simulink model "cntrl2"  (R2013a)
settings: Solver=ode45  StartTime=0.0  StopTime=20  RelTol=1e-3
undefined symbols (not defined in the file): C, G, H, K, L1
settings Model: Creator=Daniel  LastModifiedBy=Daniel

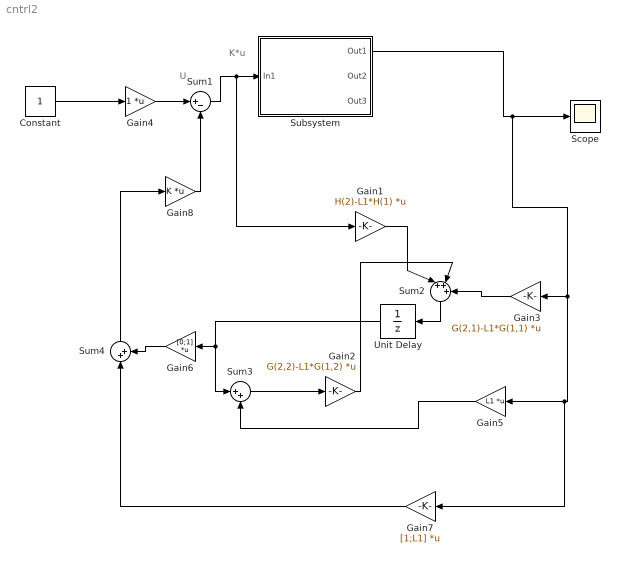
== system cntrl2 ==
  note: U
  note: K*u
  Constant : Constant
  Gain1 : Gain  Gain=H(2)-L1*H(1)  Multiplication=Matrix(K*u) (u vector)
  Gain2 : Gain  Gain=G(2,2)-L1*G(1,2)  Multiplication=Matrix(K*u) (u vector)
  Gain3 : Gain  Gain=G(2,1)-L1*G(1,1)  Multiplication=Matrix(K*u) (u vector)
  Gain4 : Gain  Multiplication=Matrix(K*u) (u vector)
  Gain5 : Gain  Gain=L1  Multiplication=Matrix(K*u) (u vector)
  Gain6 : Gain  Gain=[0;1]  Multiplication=Matrix(K*u) (u vector)
  Gain7 : Gain  Gain=[1;L1]  Multiplication=Matrix(K*u) (u vector)
  Gain8 : Gain  Gain=K  Multiplication=Matrix(K*u) (u vector)
  Scope : Scope
  Subsystem : Subsystem
      mask Display: image('b747.jpg')
  Sum1 : Sum  Inputs=|+-
  Sum2 : Sum  Inputs=|+++
  Sum3 : Sum  Inputs=|++
  Sum4 : Sum  Inputs=|++
  Unit Delay : UnitDelay  InitialCondition=4
  wires:
  Sum1/1 -> Gain1/1, Subsystem/1(In1)
  Gain4/1 -> Sum1/1
  Constant/1 -> Gain4/1
  Subsystem/1(Out1) -> Gain7/1, Gain5/1, Gain3/1, Scope/1
  Gain1/1 -> Sum2/1
  Gain3/1 -> Sum2/3
  Sum2/1 -> Unit Delay/1
  Gain2/1 -> Sum2/2
  Unit Delay/1 -> Gain6/1, Sum3/1
  Sum3/1 -> Gain2/1
  Gain5/1 -> Sum3/2
  Gain6/1 -> Sum4/2
  Gain7/1 -> Sum4/1
  Sum4/1 -> Gain8/1
  Gain8/1 -> Sum1/2

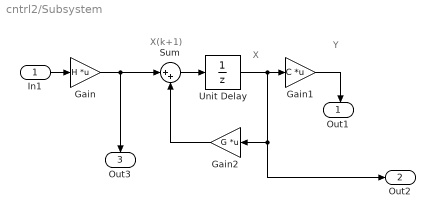
== system cntrl2/Subsystem ==
  note: X
  note: Y
  note: X(k+1)
  In1 : Inport
  Gain : Gain  Gain=H  Multiplication=Matrix(K*u) (u vector)
  Gain1 : Gain  Gain=C  Multiplication=Matrix(K*u) (u vector)
  Gain2 : Gain  Gain=G  Multiplication=Matrix(K*u) (u vector)
  Sum : Sum  Inputs=|++
  Unit Delay : UnitDelay  InitialCondition=[-1 2]
  Out1 : Outport
  Out2 : Outport  Port=2
  Out3 : Outport  Port=3
  wires:
  Gain1/1 -> Out1/1
  Unit Delay/1 -> Out2/1, Gain2/1, Gain1/1
  Gain2/1 -> Sum/2
  In1/1 -> Gain/1
  Sum/1 -> Unit Delay/1
  Gain/1 -> Sum/1, Out3/1
